simulink model "QCarModel_Free"  (R2023a)
settings: Solver=FixedStepAuto  StartTime=0.0  StopTime=20.0  FixedStep=0.1  RelTol=1e-3
values from neighbouring files (symbols this model uses):
  c = 20000    [QCarModel_Frequency_V2.m]    (also in QCarModel_Parameters.m)
  d = 1500    [QCarModel_Frequency_V2.m]    (also in QCarModel_Parameters.m)
  F = 1000    [QCarModel_Frequency_V2.m]    (also in QCarModel_Parameters.m)
  g = 981/100    (= 9.81)    [QCarModel_Frequency_V2.m]    (also in QCarModel_Parameters.m)
  m = mass(h)    [QCarModel_Frequency_V2.m]    (also in QCarModel_Parameters.m = 400)
settings Model: VariantFading=off  Creator=34140  LastModifiedBy=34140

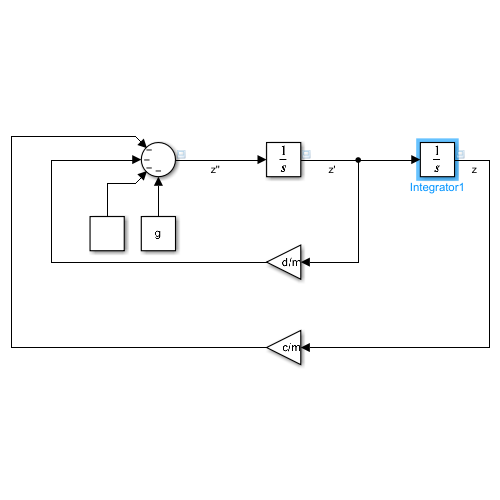
[thumbnail: Simulink's stored preview of the top-level diagram]
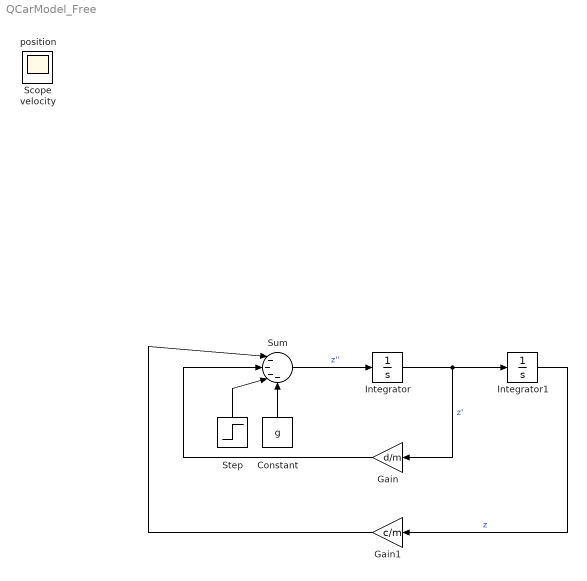
== system QCarModel_Free ==
  Constant : Constant  Value=g
  Gain : Gain  Gain=d/m
  Gain1 : Gain  Gain=c/m
  Integrator : Integrator
  Integrator1 : Integrator
  Step : Step  Time=10  After=F/m  SampleTime=0
  Sum : Sum  Inputs=|----
  Scope : Scope
  position : Scope
  velocity : Scope
  wires:
  Integrator/1 -> Gain/1, Integrator1/1  "z'"
  Sum/1 -> Integrator/1  "z''"
  Integrator1/1 -> Gain1/1  "z"
  Gain/1 -> Sum/2
  Gain1/1 -> Sum/1
  Step/1 -> Sum/3
  Constant/1 -> Sum/4
